simulink model "LED_DEMO"  (R2021a)
settings: Solver=FixedStepAuto  StartTime=0.0  StopTime=100  FixedStep=1e-3  RelTol=1e-3  EnableMultiTasking=on
libraries: frdmk64flib x3
settings Model: ExtModeTrigDuration=5  Creator=Arun Mistry  LastModifiedBy=Arun Mistry
settings OptimizationCC: EnhancedBackFolding=on  PassReuseOutputArgsAs=Individual arguments  ZeroExternalMemoryAtStartup=off  ZeroInternalMemoryAtStartup=off  MaxStackSize=64  OptimizeBlockOrder=speed  DifferentSizesBufferReuse=on  OptimizationCustomize=off  EfficientTunableParamExpr=on
settings DebuggingCC: ParameterTunabilityLossMsg=error
settings HardwareCC: ProdBitPerPointer=32  ProdBitPerSizeT=32  ProdBitPerPtrDiffT=32  ProdLargestAtomicInteger=Long  ProdLargestAtomicFloat=Double  ProdWordSize=32  ProdHWDeviceType=ARM Compatible->ARM Cortex
settings SFSimCC: MATLABDynamicMemAlloc=off
settings RTWCC: SystemTargetFile=ert.tlc  HardwareBoard=NXP FRDM-K64F  TLCOptions="-aInlineSetEventsForThisBaseRateFcn=TLC_FALSE -aSuppressMultiTaskScheduler=TLC_FALSE  -aRateBasedStepFcn=0"  TemplateMakefile=ert_default_tmf  Toolchain=GNU Tools for ARM Embedded Processors
settings CodeAppCC: ForceParamTrailComments=on  IgnoreCustomStorageClasses=off  OperatorAnnotations=on  SimulinkDataObjDesc=on  SFDataObjDesc=on  InsertBlockDesc=on
settings ERTTargetCC: ExtModeTransport=4  ExtModeMexFile=sendToCommService

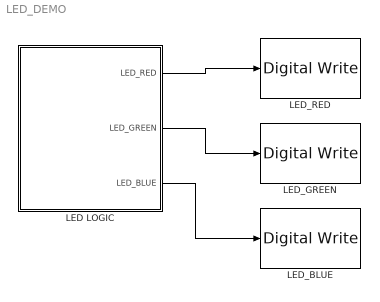
== system LED_DEMO ==
  LED LOGIC : Stateflow chart  TreatAsAtomicUnit=on
  LED_BLUE : frdmk64flib/Digital Write  Whichpin=BLUE_LED
  LED_GREEN : frdmk64flib/Digital Write  Whichpin=GREEN_LED
  LED_RED : frdmk64flib/Digital Write  Whichpin=RED_LED
  wires:
  LED LOGIC/1(LED_RED) -> LED_RED/1
  LED LOGIC/2(LED_GREEN) -> LED_GREEN/1
  LED LOGIC/3(LED_BLUE) -> LED_BLUE/1

== stateflow chart LED_DEMO/LED LOGIC ==
  state LED_RED_STATE
    entry:
    LED_BLUE = false;
    LED_RED = true;
  state LED_GREEN_STATE
    entry:
    LED_RED = false;
    LED_GREEN = true;
  state LED_BLUE_STATE
    entry:
    LED_GREEN = false;
    LED_BLUE = true;
  (default) -> LED_RED_STATE
  LED_RED_STATE -> LED_GREEN_STATE : after(5,msec)
  LED_BLUE_STATE -> LED_RED_STATE : after(5,msec)
  LED_GREEN_STATE -> LED_BLUE_STATE : after(5,msec)
  data: LED_RED output boolean; LED_GREEN output boolean; LED_BLUE output boolean
